simulink model "modules_backup"  (R2020a)
settings: Solver=VariableStepAuto  StartTime=0.0  StopTime=10.0  RelTol=1e-3
undefined symbols (not defined in the file): I_x, I_y, I_z, n
settings Model: Creator=dvdia  LastModifiedBy=dvdia

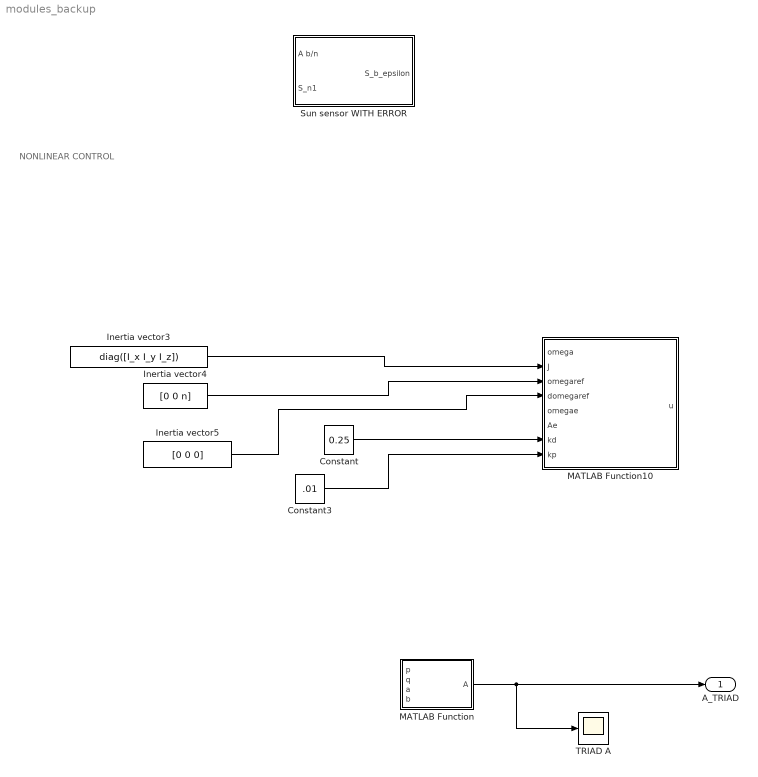
== system modules_backup ==
  note: NONLINEAR CONTROL
  Constant : Constant  Value=0.25
  Constant3 : Constant  Value=.01
  Inertia vector3 : Constant  Description=Inertia vector containing the inertias of the spacecraft in a PRINCIPAL AXIS REFERENCE SYSTEM  Value=diag([I_x I_y I_z])
  Inertia vector4 : Constant  Description=Inertia vector containing the inertias of the spacecraft in a PRINCIPAL AXIS REFERENCE SYSTEM  Value=[0 0 n]
  Inertia vector5 : Constant  Description=Inertia vector containing the inertias of the spacecraft in a PRINCIPAL AXIS REFERENCE SYSTEM  Value=[0 0 0]
  MATLAB Function : MATLAB Function  TreatAsAtomicUnit=on
  MATLAB Function10 : MATLAB Function  TreatAsAtomicUnit=on
  Sun sensor	WITH ERROR : Subsystem
  TRIAD A : Scope
  A_TRIAD : Outport
  wires:
  ? -> MATLAB Function10/1(omega)  "omega_b_OBS"
  ? -> MATLAB Function10/5(omegae)
  Constant/1 -> MATLAB Function10/7(kd)
  Constant3/1 -> MATLAB Function10/8(kp)
  Inertia vector5/1 -> MATLAB Function10/4(domegaref)
  Inertia vector4/1 -> MATLAB Function10/3(omegaref)
  Inertia vector3/1 -> MATLAB Function10/2(J)
  MATLAB Function/1(A) -> TRIAD A/1, A_TRIAD/1
  ? -> MATLAB Function/4(b)
  ? -> MATLAB Function/1(p)  "Sun sensor"
  ? -> MATLAB Function/2(q)  "EARTH sensor"
  ? -> MATLAB Function/3(a)

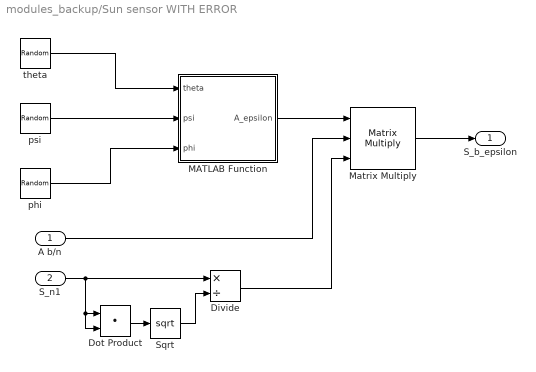
== system modules_backup/Sun sensor	WITH ERROR ==
  A b/n : Inport
  S_n1 : Inport  Port=2
  Divide : Product  Inputs=*/
  Dot Product : DotProduct  InputSameDT=on  OutDataTypeStr=Inherit: Inherit via internal rule
  MATLAB Function : MATLAB Function  TreatAsAtomicUnit=on
  Matrix Multiply : Product  Inputs=3  Multiplication=Matrix(*)
  Sqrt : Sqrt  SaturateOnIntegerOverflow=on
  phi : RandomNumber  Variance=deg2rad(1/30^2)  SampleTime=0.1
  psi : RandomNumber  Variance=deg2rad(1/30^2)  SampleTime=0.1
  theta : RandomNumber  Variance=deg2rad(1/30^2)  SampleTime=0.1
  S_b_epsilon : Outport
  wires:
  theta/1 -> MATLAB Function/1(theta)
  psi/1 -> MATLAB Function/2(psi)
  phi/1 -> MATLAB Function/3(phi)
  MATLAB Function/1(A_epsilon) -> Matrix Multiply/1
  Matrix Multiply/1 -> S_b_epsilon/1
  A b/n/1 -> Matrix Multiply/2
  Divide/1 -> Matrix Multiply/3
  S_n1/1 -> Divide/1, Dot Product/2, Dot Product/1
  Dot Product/1 -> Sqrt/1
  Sqrt/1 -> Divide/2

== matlab function modules_backup/Sun sensor	WITH ERROR/MATLAB Function ==
  data: theta input; A_epsilon output; psi input; phi input
function A_epsilon = error_matrix(theta, psi, phi)

%% Generate a random error matrix for the Sun Sensor (Lab 7)

A_epsilon = [ cos(psi)*cos(theta) cos(psi)*sin(theta)*sin(phi)+sin(psi)*cos(phi) -cos(psi)*sin(theta)*cos(phi)+sin(psi)*sin(phi)
            -sin(psi)*cos(theta)  -sin(psi)*sin(theta)*sin(phi) + cos(psi)*cos(phi) sin(psi)*sin(theta)*cos(phi) + cos(psi)*sin(phi)
            sin(theta)            -cos(theta)*sin(phi)          cos(theta)*cos(phi)];

== matlab function modules_backup/MATLAB Function10 ==
  data: omega input; u output; J input; omegaref input; domegaref input; omegae input; Ae input; kd input; kp input
function u = NONLINCONTROL(omega,J,omegaref,domegaref,omegae,Ae,kd,kp)

skewSymm = zeros(3);
skewSymm = Ae' - Ae;
skewSymm_invhat = [-skewSymm(2,3) skewSymm(1,3) -skewSymm(1,2)]';

% u = cross(omega,J*omega) - kd*omegae - kp*J*(Ae'-Ae)
u = cross(omega,J*omega) - kd*omegae - kp*skewSymm_invhat + ...
    J*(Ae*domegaref -cross(omegae,Ae*omegaref));

== matlab function modules_backup/MATLAB Function ==
  data: p input; A output; q input; a input; b input
function A = TRIAD(p,q,a,b)

s1 = p;
s2 = cross(p,q)/norm(cross(p,q));
s3 = cross(p,s2);

v1 = a;
v2 = cross(a,b)/norm(cross(a,b));
v3 = cross(a,v2);

S = [s1 s2 s3];
V = [v1 v2 v3];

A = S*(V');
